simulink model "V2_Modell_RLC"  (R2022b)
settings: Solver=ode3  StartTime=0.0  StopTime=Zeit(end)  FixedStep=0.000001  RelTol=1e-3
values from neighbouring files (symbols this model uses):
  den = [(C*R_V*L) (C*R_V*R_L+R_V*L/R_D+L) (R_V+R_L+R_V*R_L/R_D)]    [V2_Parameter_RLC_gemessen.m]    (also in V2_Parameter_RLC_nominal.m; V2_Parameter_RLC_optimiert.m)
  num = [L R_L]    [V2_Parameter_RLC_gemessen.m]    (also in V2_Parameter_RLC_nominal.m; V2_Parameter_RLC_optimiert.m)
settings Model: Creator=Patrick  LastModifiedBy=Patrick

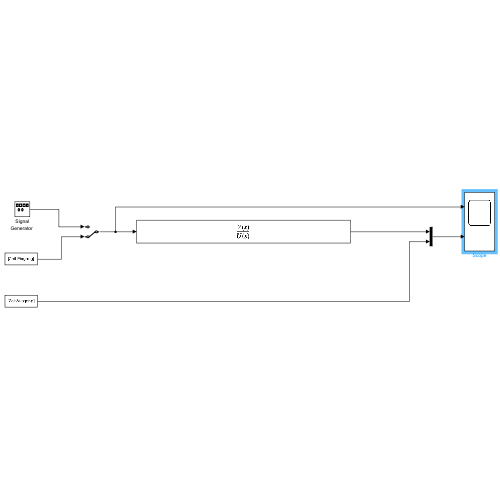
[thumbnail: Simulink's stored preview of the top-level diagram]
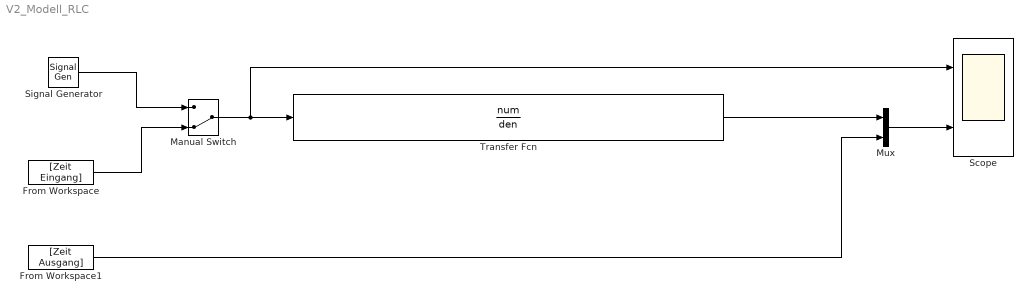
== system V2_Modell_RLC ==
  From Workspace : FromWorkspace  VariableName=[Zeit Eingang]
  From Workspace1 : FromWorkspace  VariableName=[Zeit Ausgang]
  Manual Switch : ManualSwitch  CurrentSetting=0
  Mux : Mux  Inputs=2
  Scope : Scope  NumInputPorts=2
  "Signal Generator " : SignalGenerator  Units=rad/sec
  Transfer Fcn : TransferFcn  Numerator=num  Denominator=den
  wires:
  From Workspace/1 -> Manual Switch/2
  "Signal Generator "/1 -> Manual Switch/1
  Manual Switch/1 -> Scope/1, Transfer Fcn/1
  Transfer Fcn/1 -> Mux/1
  Mux/1 -> Scope/2
  From Workspace1/1 -> Mux/2
